simulink model "simulink_ClosedLoopPID"  (Simulink 7.8)
settings: Solver=FixedStepDiscrete  SolverMode=SingleTasking  StartTime=0.0  StopTime=N*II  RelTol=1e-3
PreLoadFcn:
  | N = 1024
  | 
  | II=37+1
  | 
  |  Kp = 35.4
  |  Ki = 102
  | Kd = 0.292
  | Tf = 0.0433
  | Ts = 0.01
  | MAX_VAL  = 1024%64
  | C  = -0.7931   % derivation constant
  | Gd =  6.0324  % Derivation gain
  | Gp = 35.3675 % Proportional gain
  | Gi =  0.5112   % Integration gain
  | max_clip =   MAX_VAL-1
  | min_clip =  -MAX_VAL
StopFcn:
  | clc;
  | diff_y = simout_ref_y - simout_y;
  | figure; plot(diff_y); grid; title 'DIFF Y'
  | diff_yi = simout_ref_yi - simout_yi;
  | figure; plot(diff_yi); grid; title 'DIFF Yi'
  | diff_yd = simout_ref_yd - simout_yd;
  | figure; plot(diff_yd); grid; title 'DIFF Yd'
settings Model: Creator=danieleb  LastModifiedBy=danieleb
settings DebuggingCC: AlgebraicLoopMsg=none

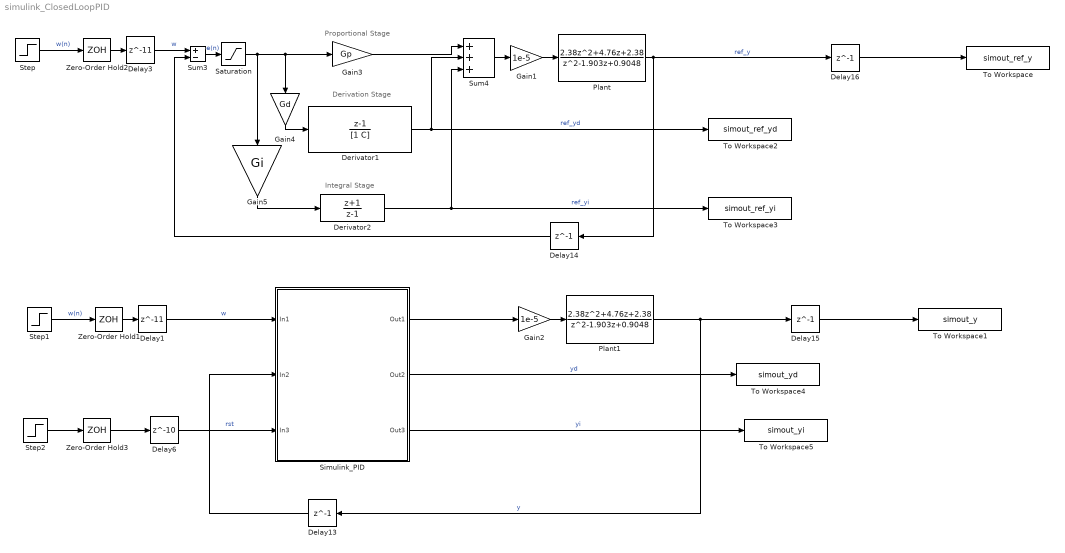
== system simulink_ClosedLoopPID ==
  note: Integral Stage
  note: Derivation Stage
  note: Proportional Stage
  Delay1 : Delay  DelayLength=11
  Delay{13..16} (4 alike) : Delay  DelayLength=1
  Delay3 : Delay  DelayLength=11
  Delay6 : Delay  DelayLength=10
  Derivator1 : DiscreteTransferFcn  Numerator=[1 -1]  Denominator=[1 C]  SampleTime=II
  Derivator2 : DiscreteTransferFcn  Numerator=[1 1]  Denominator=[1 -1]  SampleTime=II  SaturateOnIntegerOverflow=on
  Gain1 : Gain  Gain=1e-5
  Gain2 : Gain  Gain=1e-5
  Gain3 : Gain  Gain=Gp
  Gain4 : Gain  Gain=Gd
  Gain5 : Gain  Gain=Gi
  Plant : DiscreteTransferFcn  Numerator=[2.38 4.76 2.38]  Denominator=[1 -1.903 0.9048]  SampleTime=II
  Plant1 : DiscreteTransferFcn  Numerator=[2.38 4.76 2.38]  Denominator=[1 -1.903 0.9048]  SampleTime=II
  Saturation : Saturate  UpperLimit=max_clip  LowerLimit=min_clip
  Simulink_PID : Subsystem
  Step : Step  After=10  SampleTime=II
  Step1 : Step  After=10  SampleTime=II
  Step2 : Step  Before=1  After=0  SampleTime=II
  Sum3 : Sum  Inputs=+-  SampleTime=II
  Sum4 : Sum  Inputs=+++  SampleTime=II
  To Workspace : ToWorkspace  VariableName=simout_ref_y  SampleTime=-1  SaveFormat=Array
  To Workspace1 : ToWorkspace  VariableName=simout_y  SampleTime=-1  SaveFormat=Array
  To Workspace2 : ToWorkspace  VariableName=simout_ref_yd  SampleTime=-1  SaveFormat=Array
  To Workspace3 : ToWorkspace  VariableName=simout_ref_yi  SampleTime=-1  SaveFormat=Array
  To Workspace4 : ToWorkspace  VariableName=simout_yd  SampleTime=-1  SaveFormat=Array
  To Workspace5 : ToWorkspace  VariableName=simout_yi  SampleTime=-1  SaveFormat=Array
  Zero-Order Hold1 : ZeroOrderHold  SampleTime=II
  Zero-Order Hold2 : ZeroOrderHold  SampleTime=II
  Zero-Order Hold3 : ZeroOrderHold  SampleTime=II
  wires:
  Step/1 -> Zero-Order Hold2/1  "w(n)"
  Sum4/1 -> Gain1/1
  Gain3/1 -> Sum4/1
  Gain5/1 -> Derivator2/1
  Gain4/1 -> Derivator1/1
  Sum3/1 -> Saturation/1  "e(n)"
  Plant/1 -> Delay14/1, Delay16/1  "ref_y"
  Derivator1/1 -> Sum4/2, To Workspace2/1  "ref_yd"
  Derivator2/1 -> Sum4/3, To Workspace3/1  "ref_yi"
  Gain1/1 -> Plant/1
  Delay3/1 -> Sum3/1  "w"
  Zero-Order Hold2/1 -> Delay3/1
  Gain2/1 -> Plant1/1
  Simulink_PID/1(Out1) -> Gain2/1
  Simulink_PID/2(Out2) -> To Workspace4/1  "yd"
  Plant1/1 -> Delay13/1, Delay15/1  "y"
  Step1/1 -> Zero-Order Hold1/1  "w(n)"
  Delay1/1 -> Simulink_PID/1(In1)  "w"
  Zero-Order Hold1/1 -> Delay1/1
  Simulink_PID/3(Out3) -> To Workspace5/1  "yi"
  Step2/1 -> Zero-Order Hold3/1
  Zero-Order Hold3/1 -> Delay6/1
  Delay6/1 -> Simulink_PID/3(In3)  "rst"
  Saturation/1 -> Gain5/1, Gain3/1, Gain4/1
  Delay13/1 -> Simulink_PID/2(In2)
  Delay14/1 -> Sum3/2
  Delay15/1 -> To Workspace1/1
  Delay16/1 -> To Workspace/1

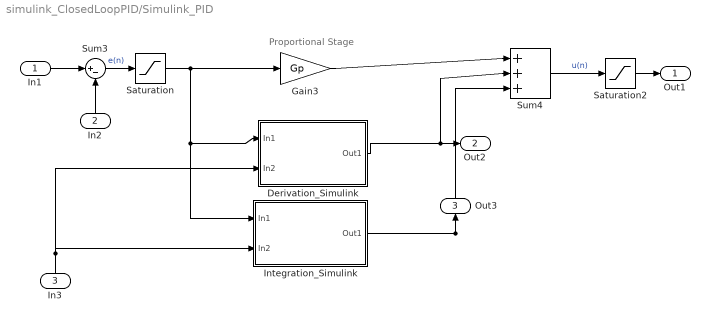
== system simulink_ClosedLoopPID/Simulink_PID ==
  note: Proportional Stage
  In1 : Inport
  In2 : Inport  Port=2
  In3 : Inport  Port=3
  Derivation_Simulink : Subsystem
  Gain3 : Gain  Gain=Gp
  Integration_Simulink : Subsystem
  Saturation : Saturate  UpperLimit=max_clip  LowerLimit=min_clip
  Saturation2 : Saturate  UpperLimit=max_clip  LowerLimit=min_clip
  Sum3 : Sum  Inputs=|+-
  Sum4 : Sum  Inputs=|+++
  Out1 : Outport
  Out2 : Outport  Port=2
  Out3 : Outport  Port=3
  wires:
  Gain3/1 -> Sum4/1
  Sum3/1 -> Saturation/1  "e(n)"
  Sum4/1 -> Saturation2/1  "u(n)"
  Saturation/1 -> Gain3/1, Derivation_Simulink/1(In1), Integration_Simulink/1(In1)
  Derivation_Simulink/1(Out1) -> Sum4/2, Out2/1
  Integration_Simulink/1(Out1) -> Sum4/3, Out3/1
  In1/1 -> Sum3/1
  In2/1 -> Sum3/2
  In3/1 -> Integration_Simulink/2(In2), Derivation_Simulink/2(In2)
  Saturation2/1 -> Out1/1

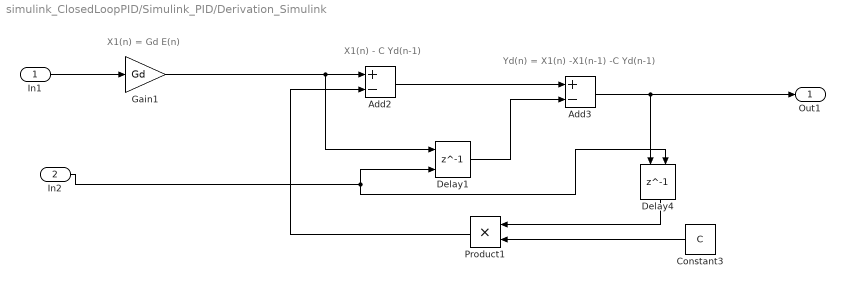
== system simulink_ClosedLoopPID/Simulink_PID/Derivation_Simulink ==
  note: X1(n) - C Yd(n-1)
  note: Yd(n) = X1(n) -X1(n-1) -C Yd(n-1)
  note: X1(n) = Gd E(n)
  In1 : Inport
  In2 : Inport  Port=2
  Add2 : Sum  Inputs=+-
  Add3 : Sum  Inputs=+-
  Constant3 : Constant  Value=C  OutDataTypeStr=single  SampleTime=II
  Delay1 : Delay  DelayLength=1  ExternalReset=Level hold
      settings: InputPortMap=u0,r5
  Delay4 : Delay  DelayLength=1  ExternalReset=Level hold
      settings: InputPortMap=u0,r5
  Gain1 : Gain  Gain=Gd
  Product1 : Product  RndMeth=Zero
  Out1 : Outport
  wires:
  In1/1 -> Gain1/1
  Delay1/1 -> Add3/2
  Add2/1 -> Add3/1
  Add3/1 -> Delay4/1, Out1/1
  Constant3/1 -> Product1/2
  Product1/1 -> Add2/2
  Delay4/1 -> Product1/1
  In2/1 -> Delay1/2, Delay4/2
  Gain1/1 -> Add2/1, Delay1/1

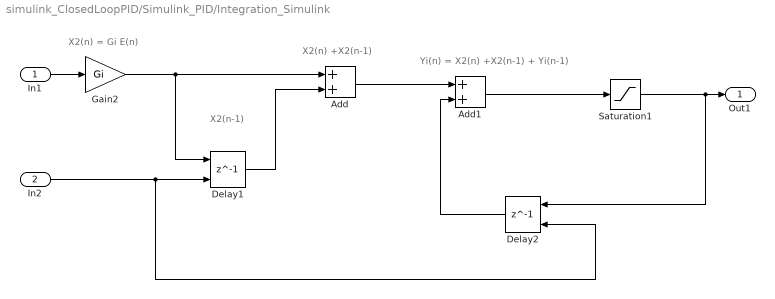
== system simulink_ClosedLoopPID/Simulink_PID/Integration_Simulink ==
  note: X2(n) = Gi E(n)
  note: X2(n) +X2(n-1)
  note: X2(n-1)
  note: Yi(n) = X2(n) +X2(n-1) + Yi(n-1)
  In1 : Inport
  In2 : Inport  Port=2
  Add : Sum
  Add1 : Sum
  Delay1 : Delay  DelayLength=1  ExternalReset=Level hold
      settings: InputPortMap=u0,r5
  Delay2 : Delay  DelayLength=1  ExternalReset=Level hold
      settings: InputPortMap=u0,r5
  Gain2 : Gain  Gain=Gi
  Saturation1 : Saturate  UpperLimit=max_clip  LowerLimit=min_clip
  Out1 : Outport
  wires:
  Add/1 -> Add1/1
  Add1/1 -> Saturation1/1
  Gain2/1 -> Add/1, Delay1/1
  Delay1/1 -> Add/2
  Saturation1/1 -> Out1/1, Delay2/1
  In1/1 -> Gain2/1
  Delay2/1 -> Add1/2
  In2/1 -> Delay1/2, Delay2/2
